simulink subsystem "visualization"  (R2024b)
settings: Solver=VariableStepAuto  StartTime=0.0  StopTime=10.0  RelTol=1e-3
values from neighbouring files (symbols this model uses):
  alt = [-0.000386 -0.000185 1.575e-05 0.001 0.009 0.025 0.054 0.095 0.149 0.216 0.296 0.389 ... (1300 elements, 1300x1)]    [barrowaman.mat]
  angle_vert_deg = [5 5 5 5 5 5 5 5 5 5 5 5 ... (1300 elements, 1300x1)]    [barrowaman.mat]
  crossrange = [3.38e-05 1.622e-05 1.378e-06 0.0001312 0.0007491 0.002 0.005 0.008 0.013 0.019 0.026 0.034 ... (1300 elements, 1300x1)]    [barrowaman.mat]
  sim_time = [0.01 0.02 0.03 0.04 0.05 0.06 0.07 0.08 0.09 0.1 0.11 0.12 ... (1300 elements, 1300x1)]    [barrowaman.mat]
  vel_ver = [-0.077 -0.037 0.003 0.294 1.119 2.251 3.462 4.75 6.068 7.366 8.647 9.915 ... (1300 elements, 1300x1)]    [barrowaman.mat]
libraries: aerolibanim x1, simulink_extras x1
settings Model: Creator=joedo  LastModifiedBy=trist

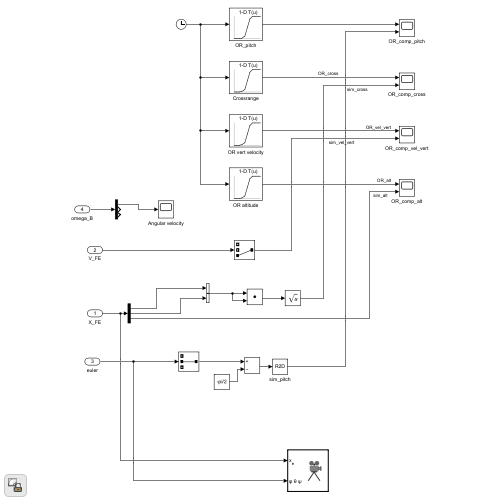
[thumbnail: Simulink's stored preview of the top-level diagram]
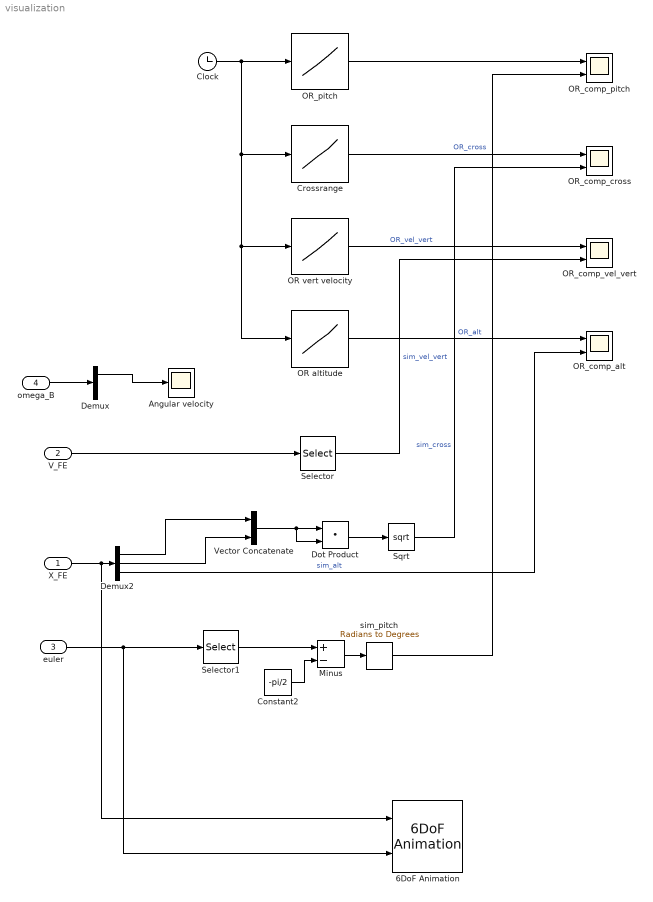
== system visualization ==
  X_FE : Inport
  V_FE : Inport  Port=2
  euler : Inport  Port=3
  omega_B : Inport  Port=4
  6DoF Animation : aerolibanim/6DoF Animation  u1=[0 400 -200 200 0 4000]  u2=0.1  u3=100  u4=[4000 0 -5000]  u5=Fixed position  u6=[2000 500 3150]  u7=10  u8=off
  Angular velocity : Scope
  Clock : Clock
  Constant2 : Constant  Value=-pi/2
  Crossrange : Lookup_n-D  NumberOfTableDimensions=1  BreakpointsForDimension1=sim_time  Table=crossrange  InternalRulePriority=Speed  RndMeth=Simplest
  Demux : Demux  Outputs=3
  Demux2 : Demux  Outputs=3
  Dot Product : DotProduct  OutDataTypeStr=Inherit: Inherit via internal rule
  Minus : Sum  Inputs=+-
  OR altitude : Lookup_n-D  NumberOfTableDimensions=1  BreakpointsForDimension1=sim_time  Table=alt  InternalRulePriority=Speed  RndMeth=Simplest
  OR vert velocity : Lookup_n-D  NumberOfTableDimensions=1  BreakpointsForDimension1=sim_time  Table=vel_ver  InternalRulePriority=Speed  RndMeth=Simplest
  OR_comp_alt : Scope  NumInputPorts=2
  OR_comp_cross : Scope  NumInputPorts=2
  OR_comp_pitch : Scope  NumInputPorts=2
  OR_comp_vel_vert : Scope  NumInputPorts=2
  OR_pitch : Lookup_n-D  NumberOfTableDimensions=1  BreakpointsForDimension1=sim_time  Table=angle_vert_deg  InternalRulePriority=Speed  RndMeth=Simplest
  Selector : Selector  InputPortWidth=3  IndexOptions=Index vector (dialog)  Indices=[3]  OutputSizes=1
  Selector1 : Selector  InputPortWidth=3  IndexOptions=Index vector (dialog)  Indices=[2]  OutputSizes=1
  Sqrt : Sqrt
  Vector Concatenate : Concatenate
  sim_pitch : simulink_extras/Transformations/Radians to Degrees
  wires:
  Constant2/1 -> Minus/2
  Vector Concatenate/1 -> Dot Product/1, Dot Product/2
  Demux2/1 -> Vector Concatenate/1
  Crossrange/1 -> OR_comp_cross/1  "OR_cross"
  Clock/1 -> OR_pitch/1, OR altitude/1, OR vert velocity/1, Crossrange/1
  Demux2/2 -> Vector Concatenate/2
  OR_pitch/1 -> OR_comp_pitch/1
  Minus/1 -> sim_pitch/1
  sim_pitch/1 -> OR_comp_pitch/2
  OR altitude/1 -> OR_comp_alt/1  "OR_alt"
  Demux2/3 -> OR_comp_alt/2  "sim_alt"
  Selector/1 -> OR_comp_vel_vert/2  "sim_vel_vert"
  Dot Product/1 -> Sqrt/1
  Sqrt/1 -> OR_comp_cross/2  "sim_cross"
  euler/1 -> Selector1/1, 6DoF Animation/2
  OR vert velocity/1 -> OR_comp_vel_vert/1  "OR_vel_vert"
  X_FE/1 -> Demux2/1, 6DoF Animation/1
  V_FE/1 -> Selector/1
  Selector1/1 -> Minus/1
  omega_B/1 -> Demux/1
  Demux/1 -> Angular velocity/1
